simulink model "Stage_4_6_CAN_Fault_Diagnostics_Combined_fault"  (R2025a)
settings: Solver=VariableStepAuto  StartTime=0.0  StopTime=12  RelTol=1e-3
libraries: SignalEditorBlockLib x13, canmsglib x9, simulink x5
settings Model: Creator=sitam  LastModifiedBy=sitam

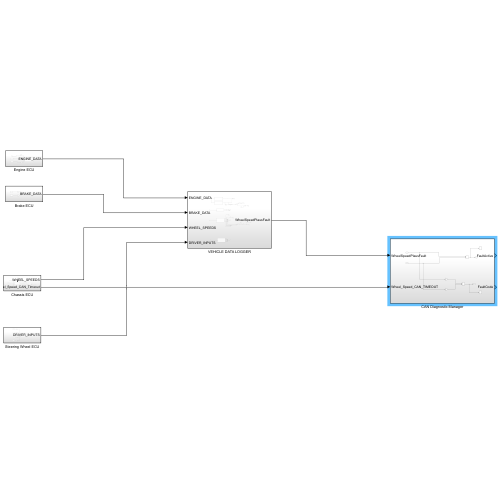
[thumbnail: Simulink's stored preview of the top-level diagram]
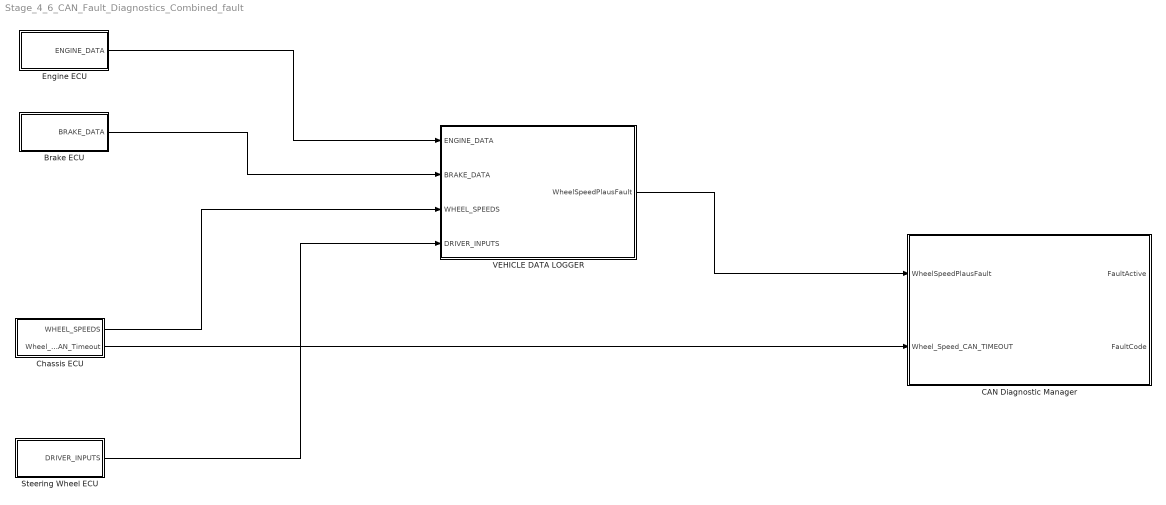
== system Stage_4_6_CAN_Fault_Diagnostics_Combined_fault ==
  Brake ECU : Subsystem
  CAN Diagnostic Manager : Subsystem
  Chassis ECU : Subsystem
  Engine ECU : Subsystem
  Steering Wheel ECU : Subsystem
  VEHICLE DATA LOGGER : Subsystem
  wires:
  Engine ECU/1(ENGINE_DATA) -> VEHICLE DATA LOGGER/1(ENGINE_DATA)
  Brake ECU/1(BRAKE_DATA) -> VEHICLE DATA LOGGER/2(BRAKE_DATA)
  Chassis ECU/1(WHEEL_SPEEDS) -> VEHICLE DATA LOGGER/3(WHEEL_SPEEDS)
  Steering Wheel ECU/1(DRIVER_INPUTS) -> VEHICLE DATA LOGGER/4(DRIVER_INPUTS)
  VEHICLE DATA LOGGER/1(WheelSpeedPlausFault) -> CAN Diagnostic Manager/1(WheelSpeedPlausFault)
  Chassis ECU/2(Wheel_Speed_CAN_Timeout) -> CAN Diagnostic Manager/2(Wheel_Speed_CAN_TIMEOUT)

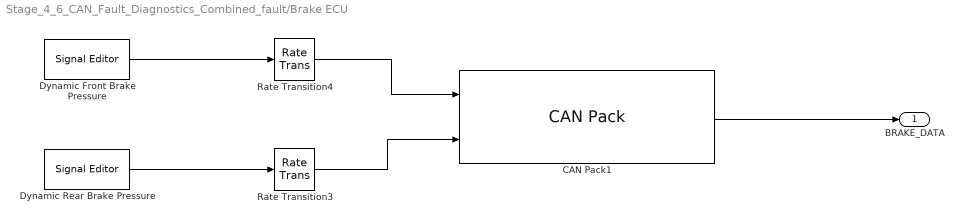
== system Stage_4_6_CAN_Fault_Diagnostics_Combined_fault/Brake ECU ==
  CAN Pack1 : canmsglib/CAN Pack  CANdbFile=C:\Users\sitam\OneDrive\Projects\CAN Bus Project\MotorsportCAN.dbc  MsgList=BRAKE_DATA  MsgName=BRAKE_DATA  MsgIDType=Standard (11-bit identifier)  MsgIdentifier=512  CANIDInput=off  MsgLength=8  Remote=off  ApplyMinMax=off  BusOutput=off  SignalInfo={'FrontBrakePressure','0','16','LE','unsigned','Standard','0','0.01','0','0','200';'RearBrakePressure','16','16','LE','unsigned','Standard','0','0.01','0','0','200'}
      settings: LibrarySourceBlock=canlib/CAN Pack  DataFormat=CANdb specified signals
  Dynamic Front Brake Pressure : SignalEditorBlockLib/Signal Editor  FileName=3_frontbrake.mat  ActiveScenario=Scenario  ActiveSignal=Signal 1  IsBus=off  OutputBusObjectStr=Bus: BusObject  SampleTime=0  ZeroCross=off  OutputAfterFinalValue=Setting to zero  Unit=inherit  PreserveSignalName=on  ApplySigPropsToAllScenarios=on  ApplySigPropsToAllSignals=off  SignalPropertySource=Dialog parameters
  Dynamic Rear Brake Pressure : SignalEditorBlockLib/Signal Editor  FileName=3_rearbrake.mat  ActiveScenario=Scenario  ActiveSignal=Signal 1  IsBus=off  OutputBusObjectStr=Bus: BusObject  SampleTime=0  ZeroCross=off  OutputAfterFinalValue=Setting to zero  Unit=inherit  PreserveSignalName=on  ApplySigPropsToAllScenarios=on  ApplySigPropsToAllSignals=off  SignalPropertySource=Dialog parameters
  Rate Transition3 : RateTransition  OutPortSampleTime=0.01
  Rate Transition4 : RateTransition  OutPortSampleTime=0.01
  BRAKE_DATA : Outport
  wires:
  Rate Transition4/1 -> CAN Pack1/1
  Rate Transition3/1 -> CAN Pack1/2
  CAN Pack1/1 -> BRAKE_DATA/1
  Dynamic Front Brake Pressure/1 -> Rate Transition4/1
  Dynamic Rear Brake Pressure/1 -> Rate Transition3/1

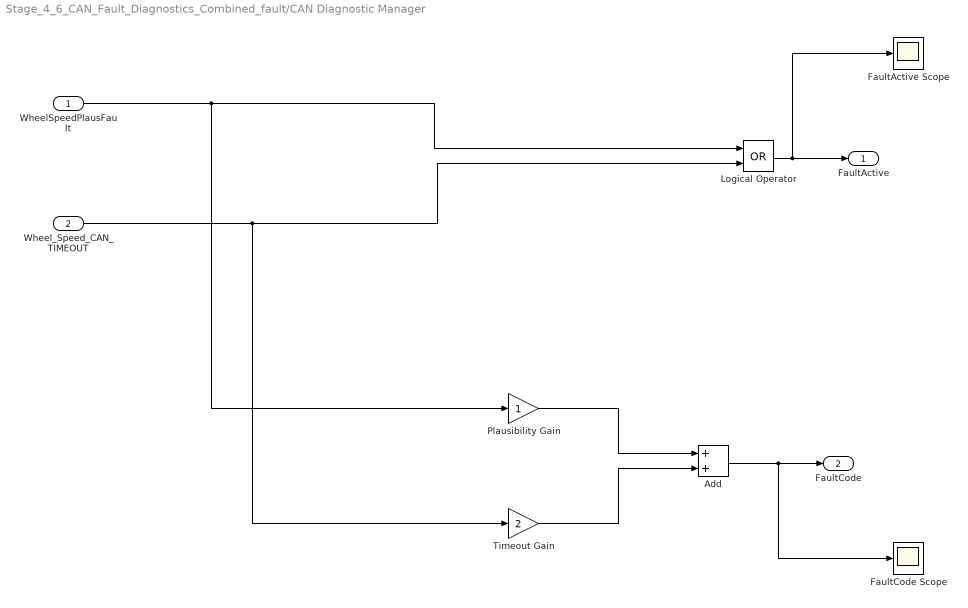
== system Stage_4_6_CAN_Fault_Diagnostics_Combined_fault/CAN Diagnostic Manager ==
  WheelSpeedPlausFault : Inport
  Wheel_Speed_CAN_TIMEOUT : Inport  Port=2
  Add : Sum
  FaultActive Scope : Scope
      settings: ActiveDisplayYMinimum=-0.12499999999999997  ActiveDisplayYMaximum=1.125
  FaultCode Scope : Scope
      settings: ActiveDisplayYMinimum=-0.37499999999999989  ActiveDisplayYMaximum=3.375  DataLoggingVariableName=ScopeData2
  Logical Operator : Logic  Operator=OR  AllPortsSameDT=off  OutDataTypeStr=boolean
  Plausibility Gain : Gain
  Timeout Gain : Gain  Gain=2
  FaultActive : Outport
  FaultCode : Outport  Port=2
  wires:
  WheelSpeedPlausFault/1 -> Plausibility Gain/1, Logical Operator/1
  Wheel_Speed_CAN_TIMEOUT/1 -> Timeout Gain/1, Logical Operator/2
  Logical Operator/1 -> FaultActive Scope/1, FaultActive/1
  Plausibility Gain/1 -> Add/1
  Timeout Gain/1 -> Add/2
  Add/1 -> FaultCode Scope/1, FaultCode/1

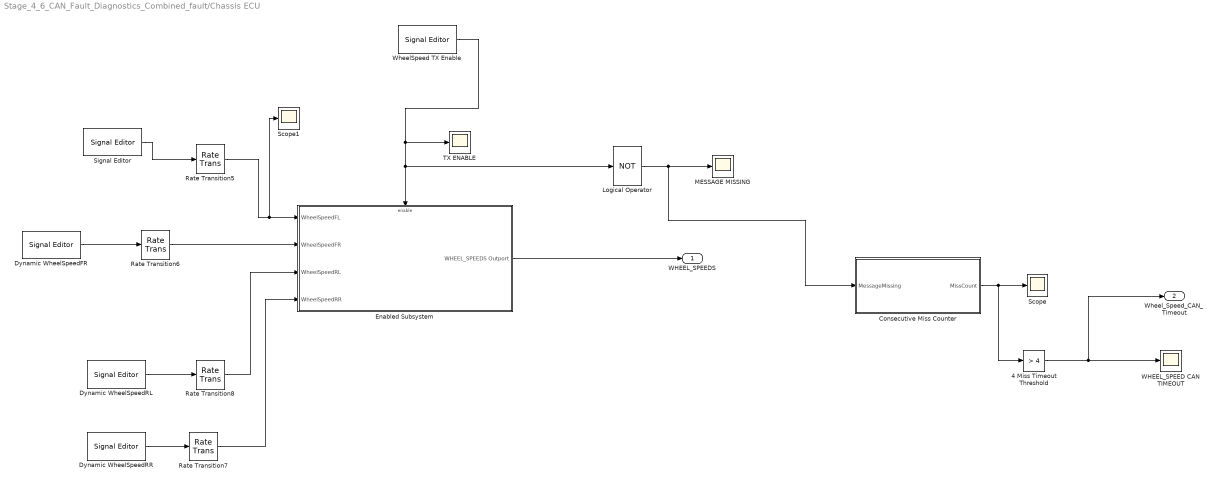
== system Stage_4_6_CAN_Fault_Diagnostics_Combined_fault/Chassis ECU ==
  4 Miss Timeout Threshold : simulink/Logic and Bit Operations/Compare To Constant  relop=>  const=4  OutDataTypeStr=boolean
  Consecutive Miss Counter : Subsystem
  Dynamic WheelSpeedFR : SignalEditorBlockLib/Signal Editor  FileName=3_WheelSpeedFR.mat  ActiveScenario=Scenario  ActiveSignal=Signal 1  IsBus=off  OutputBusObjectStr=Bus: BusObject  SampleTime=0  ZeroCross=off  OutputAfterFinalValue=Setting to zero  Unit=inherit  PreserveSignalName=on  ApplySigPropsToAllScenarios=on  ApplySigPropsToAllSignals=off  SignalPropertySource=Dialog parameters
  Dynamic WheelSpeedRL : SignalEditorBlockLib/Signal Editor  FileName=3_WheelSpeedRL.mat  ActiveScenario=Scenario  ActiveSignal=Signal 1  IsBus=off  OutputBusObjectStr=Bus: BusObject  SampleTime=0  ZeroCross=off  OutputAfterFinalValue=Setting to zero  Unit=inherit  PreserveSignalName=on  ApplySigPropsToAllScenarios=on  ApplySigPropsToAllSignals=off  SignalPropertySource=Dialog parameters
  Dynamic WheelSpeedRR : SignalEditorBlockLib/Signal Editor  FileName=3_WheelSpeedRR.mat  ActiveScenario=Scenario  ActiveSignal=Signal 1  IsBus=off  OutputBusObjectStr=Bus: BusObject  SampleTime=0  ZeroCross=off  OutputAfterFinalValue=Setting to zero  Unit=inherit  PreserveSignalName=on  ApplySigPropsToAllScenarios=on  ApplySigPropsToAllSignals=off  SignalPropertySource=Dialog parameters
  Enabled Subsystem : Subsystem  TreatAsAtomicUnit=on
  Logical Operator : Logic  Operator=NOT  AllPortsSameDT=off  OutDataTypeStr=boolean
  MESSAGE MISSING : Scope
      settings: ActiveDisplayYMinimum=-0.16704928841560512  ActiveDisplayYMaximum=1.2799819615843948  DataLoggingVariableName=ScopeData2
  Rate Transition{5..8} (4 alike) : RateTransition  OutPortSampleTime=0.005
  Scope : Scope
      settings: ActiveDisplayYMinimum=-50.124999999999986  ActiveDisplayYMaximum=451.125  DataLoggingVariableName=ScopeData3
  Scope1 : Scope
      settings: ActiveDisplayYMinimum=7.5000000000000071  ActiveDisplayYMaximum=332.5  DataLoggingVariableName=ScopeData5
  Signal Editor : SignalEditorBlockLib/Signal Editor  FileName=4_6WheelspeedFL.mat  ActiveScenario=Scenario  ActiveSignal=Signal 1  IsBus=off  OutputBusObjectStr=Bus: BusObject  SampleTime=0  ZeroCross=off  OutputAfterFinalValue=Setting to zero  Unit=inherit  PreserveSignalName=on  ApplySigPropsToAllScenarios=on  ApplySigPropsToAllSignals=off  SignalPropertySource=Dialog parameters
  TX ENABLE : Scope
      settings: ActiveDisplayYMinimum=-1  ActiveDisplayYMaximum=1
  WHEEL_SPEED CAN TIMEOUT : Scope
      settings: ActiveDisplayYMinimum=-0.12499999999999997  ActiveDisplayYMaximum=1.125  DataLoggingVariableName=ScopeData4
  WheelSpeed TX Enable : SignalEditorBlockLib/Signal Editor  FileName=4_6WHEEL_SPEEDS_Tx_Enable.mat  ActiveScenario=Scenario  ActiveSignal=Signal 1  IsBus=off  OutputBusObjectStr=Bus: BusObject  SampleTime=0  ZeroCross=off  OutputAfterFinalValue=Setting to zero  Unit=inherit  PreserveSignalName=on  ApplySigPropsToAllScenarios=on  ApplySigPropsToAllSignals=off  SignalPropertySource=Dialog parameters
  WHEEL_SPEEDS : Outport
  Wheel_Speed_CAN_Timeout : Outport  Port=2
  wires:
  Rate Transition8/1 -> Enabled Subsystem/3(WheelSpeedRL)
  Enabled Subsystem/1(WHEEL_SPEEDS Outport) -> WHEEL_SPEEDS/1
  Dynamic WheelSpeedFR/1 -> Rate Transition6/1
  Dynamic WheelSpeedRL/1 -> Rate Transition8/1
  Rate Transition5/1 -> Scope1/1, Enabled Subsystem/1(WheelSpeedFL)
  Dynamic WheelSpeedRR/1 -> Rate Transition7/1
  Rate Transition7/1 -> Enabled Subsystem/4(WheelSpeedRR)
  Rate Transition6/1 -> Enabled Subsystem/2(WheelSpeedFR)
  Logical Operator/1 -> Consecutive Miss Counter/1(MessageMissing), MESSAGE MISSING/1
  Consecutive Miss Counter/1(MissCount) -> 4 Miss Timeout Threshold/1, Scope/1
  4 Miss Timeout Threshold/1 -> Wheel_Speed_CAN_Timeout/1, WHEEL_SPEED CAN TIMEOUT/1
  Signal Editor/1 -> Rate Transition5/1
  WheelSpeed TX Enable/1 -> TX ENABLE/1, Enabled Subsystem/Enable, Logical Operator/1

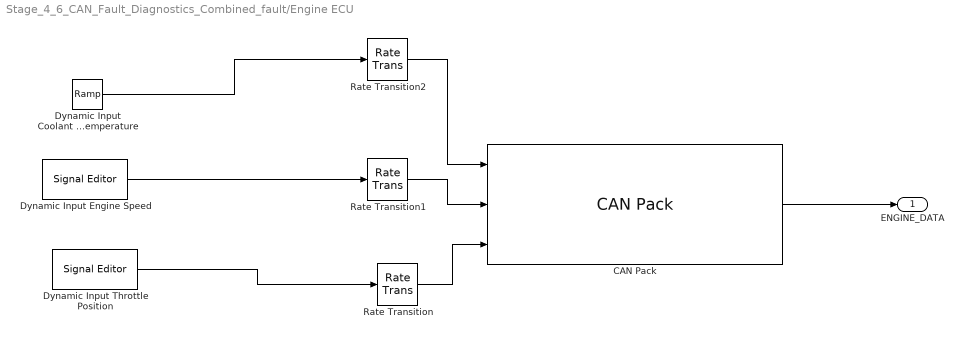
== system Stage_4_6_CAN_Fault_Diagnostics_Combined_fault/Engine ECU ==
  CAN Pack : canmsglib/CAN Pack  CANdbFile=C:\Users\sitam\OneDrive\Projects\CAN Bus Project\MotorsportCAN.dbc  MsgList=ENGINE_DATA  MsgName=ENGINE_DATA  MsgIDType=Standard (11-bit identifier)  MsgIdentifier=256  CANIDInput=off  MsgLength=8  Remote=off  ApplyMinMax=off  BusOutput=off  SignalInfo={'CoolantTemperature','24','8','LE','unsigned','Standard','0','1','-40','-40','150';'EngineSpeed','0','16','LE','unsigned','Standard','0','0.25','0','0','15000';'ThrottlePosition','16','8','LE','unsigned','Standard','0','0.4','0','0','100'}
      settings: LibrarySourceBlock=canlib/CAN Pack  DataFormat=CANdb specified signals
  Dynamic Input Coolant Temperature : simulink/Sources/Ramp  slope=1  start=0  InitialOutput=85
  Dynamic Input Engine Speed : SignalEditorBlockLib/Signal Editor  FileName=2_2-enginespeed.mat  ActiveScenario=Scenario  ActiveSignal=Signal 1  IsBus=off  OutputBusObjectStr=Bus: BusObject  SampleTime=0  ZeroCross=off  OutputAfterFinalValue=Setting to zero  Unit=inherit  PreserveSignalName=on  ApplySigPropsToAllScenarios=on  ApplySigPropsToAllSignals=off  SignalPropertySource=Dialog parameters
  Dynamic Input Throttle Position : SignalEditorBlockLib/Signal Editor  FileName=2_2-throttlepos.mat  ActiveScenario=Scenario  ActiveSignal=Signal 1  IsBus=off  OutputBusObjectStr=Bus: BusObject  SampleTime=0  ZeroCross=off  OutputAfterFinalValue=Setting to zero  Unit=inherit  PreserveSignalName=on  ApplySigPropsToAllScenarios=on  ApplySigPropsToAllSignals=off  SignalPropertySource=Dialog parameters
  Rate Transition : RateTransition  OutPortSampleTime=0.01
  Rate Transition1 : RateTransition  OutPortSampleTime=0.01
  Rate Transition2 : RateTransition  OutPortSampleTime=0.01
  ENGINE_DATA : Outport
  wires:
  CAN Pack/1 -> ENGINE_DATA/1
  Dynamic Input Coolant Temperature/1 -> Rate Transition2/1
  Rate Transition2/1 -> CAN Pack/1
  Dynamic Input Engine Speed/1 -> Rate Transition1/1
  Rate Transition1/1 -> CAN Pack/2
  Dynamic Input Throttle Position/1 -> Rate Transition/1
  Rate Transition/1 -> CAN Pack/3

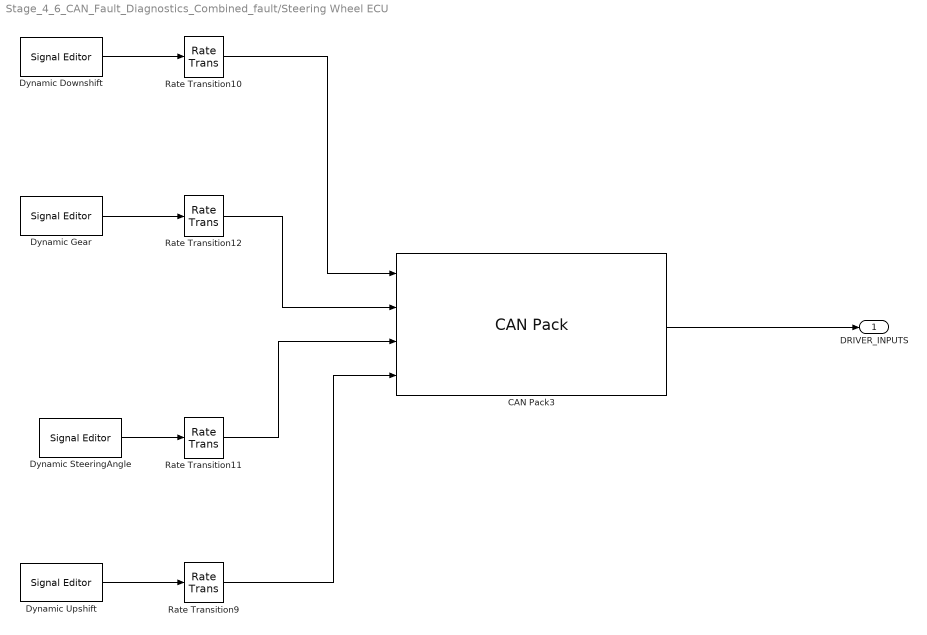
== system Stage_4_6_CAN_Fault_Diagnostics_Combined_fault/Steering Wheel ECU ==
  CAN Pack3 : canmsglib/CAN Pack  CANdbFile=C:\Users\sitam\OneDrive\Projects\CAN Bus Project\MotorsportCAN.dbc  MsgList=DRIVER_INPUTS  MsgName=DRIVER_INPUTS  MsgIDType=Standard (11-bit identifier)  MsgIdentifier=1024  CANIDInput=off  MsgLength=8  Remote=off  ApplyMinMax=off  BusOutput=off  SignalInfo={'Downshift','25','1','LE','unsigned','Standard','0','1','0','0','1';'Gear','16','3','LE','unsigned','Standard','0','1','0','0','7';'SteeringAngle','0','16','LE','signed','Standard','0','0.1','0','-540','540';'Upshift','24','1','LE','unsigned','Standard','0','1','0','0','1'}
      settings: LibrarySourceBlock=canlib/CAN Pack  DataFormat=CANdb specified signals
  Dynamic Downshift : SignalEditorBlockLib/Signal Editor  FileName=3_downshift.mat  ActiveScenario=Scenario  ActiveSignal=Signal 1  IsBus=off  OutputBusObjectStr=Bus: BusObject  SampleTime=0  ZeroCross=off  OutputAfterFinalValue=Setting to zero  Unit=inherit  PreserveSignalName=on  ApplySigPropsToAllScenarios=on  ApplySigPropsToAllSignals=off  SignalPropertySource=Dialog parameters
  Dynamic Gear : SignalEditorBlockLib/Signal Editor  FileName=3_gear.mat  ActiveScenario=Scenario  ActiveSignal=Signal 1  IsBus=off  OutputBusObjectStr=Bus: BusObject  SampleTime=0  ZeroCross=off  OutputAfterFinalValue=Setting to zero  Unit=inherit  PreserveSignalName=on  ApplySigPropsToAllScenarios=on  ApplySigPropsToAllSignals=off  SignalPropertySource=Dialog parameters
  Dynamic SteeringAngle : SignalEditorBlockLib/Signal Editor  FileName=3_steeringangle.mat  ActiveScenario=Scenario  ActiveSignal=Signal 1  IsBus=off  OutputBusObjectStr=Bus: BusObject  SampleTime=0  ZeroCross=off  OutputAfterFinalValue=Setting to zero  Unit=inherit  PreserveSignalName=on  ApplySigPropsToAllScenarios=on  ApplySigPropsToAllSignals=off  SignalPropertySource=Dialog parameters
  Dynamic Upshift : SignalEditorBlockLib/Signal Editor  FileName=3_upshift.mat  ActiveScenario=Scenario  ActiveSignal=Signal 1  IsBus=off  OutputBusObjectStr=Bus: BusObject  SampleTime=0  ZeroCross=off  OutputAfterFinalValue=Setting to zero  Unit=inherit  PreserveSignalName=on  ApplySigPropsToAllScenarios=on  ApplySigPropsToAllSignals=off  SignalPropertySource=Dialog parameters
  Rate Transition{9..12} (4 alike) : RateTransition  OutPortSampleTime=0.02
  DRIVER_INPUTS : Outport
  wires:
  Rate Transition10/1 -> CAN Pack3/1
  Dynamic Upshift/1 -> Rate Transition9/1
  Rate Transition11/1 -> CAN Pack3/3
  Dynamic SteeringAngle/1 -> Rate Transition11/1
  Rate Transition9/1 -> CAN Pack3/4
  Rate Transition12/1 -> CAN Pack3/2
  Dynamic Gear/1 -> Rate Transition12/1
  Dynamic Downshift/1 -> Rate Transition10/1
  CAN Pack3/1 -> DRIVER_INPUTS/1

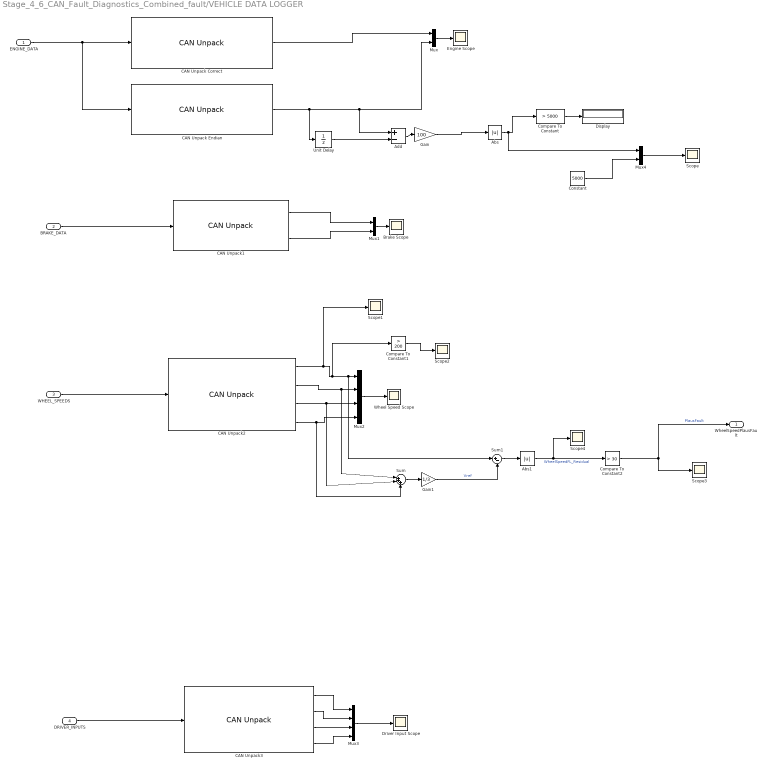
== system Stage_4_6_CAN_Fault_Diagnostics_Combined_fault/VEHICLE DATA LOGGER ==
  ENGINE_DATA : Inport
  BRAKE_DATA : Inport  Port=2
  WHEEL_SPEEDS : Inport  Port=3
  DRIVER_INPUTS : Inport  Port=4
  Abs : Abs  SaturateOnIntegerOverflow=off
  Abs1 : Abs  SaturateOnIntegerOverflow=off
  Add : Sum  Inputs=+-
  Brake Scope : Scope
      settings: ActiveDisplayYMinimum=-1  ActiveDisplayYMaximum=1  DataLoggingVariableName=ScopeData15
  CAN Unpack Correct : canmsglib/CAN Unpack  CANdbFile=C:\Users\sitam\OneDrive\Projects\CAN Bus Project\MotorsportCAN.dbc  MsgList=ENGINE_DATA  MsgName=ENGINE_DATA  MsgIDType=Standard (11-bit identifier)  MsgIdentifier=256  MsgLength=8  SignalInfo={'CoolantTemperature','24','8','LE','unsigned','Standard','0','1','-40','-40','150';'EngineSpeed','0','16','LE','unsigned','Standard','0','0.25','0','0','15000';'ThrottlePosition','16','8','LE','unsigned','Standard','0','0.4','0','0','100'}  IDPort=off  TimestampPort=off  ErrorPort=off  RemotePort=off  LengthPort=off  StatusPort=off  ApplyMinMax=off
      settings: LibrarySourceBlock=canlib/CAN Unpack  DataFormat=CANdb specified signals
  CAN Unpack Endian : canmsglib/CAN Unpack  CANdbFile=C:\Users\sitam\OneDrive\Projects\CAN Bus Project\dbc files\MotorsportCAN_Fault_Endian.dbc  MsgList=ENGINE_DATA  MsgName=ENGINE_DATA  MsgIDType=Standard (11-bit identifier)  MsgIdentifier=256  MsgLength=8  SignalInfo={'CoolantTemperature','24','8','LE','unsigned','Standard','0','1','-40','-40','150';'EngineSpeed','8','16','BE','unsigned','Standard','0','0.25','0','0','15000';'ThrottlePosition','16','8','LE','unsigned','Standard','0','0.4','0','0','100'}  IDPort=off  TimestampPort=off  ErrorPort=off  RemotePort=off  LengthPort=off  StatusPort=off  ApplyMinMax=off
      settings: LibrarySourceBlock=canlib/CAN Unpack  DataFormat=CANdb specified signals
  CAN Unpack1 : canmsglib/CAN Unpack  CANdbFile=C:\Users\sitam\OneDrive\Projects\CAN Bus Project\MotorsportCAN.dbc  MsgList=BRAKE_DATA  MsgName=BRAKE_DATA  MsgIDType=Standard (11-bit identifier)  MsgIdentifier=512  MsgLength=8  SignalInfo={'FrontBrakePressure','0','16','LE','unsigned','Standard','0','0.01','0','0','200';'RearBrakePressure','16','16','LE','unsigned','Standard','0','0.01','0','0','200'}  IDPort=off  TimestampPort=off  ErrorPort=off  RemotePort=off  LengthPort=off  StatusPort=off  ApplyMinMax=off
      settings: LibrarySourceBlock=canlib/CAN Unpack  DataFormat=CANdb specified signals
  CAN Unpack2 : canmsglib/CAN Unpack  CANdbFile=C:\Users\sitam\OneDrive\Projects\CAN Bus Project\MotorsportCAN.dbc  MsgList=WHEEL_SPEEDS  MsgName=WHEEL_SPEEDS  MsgIDType=Standard (11-bit identifier)  MsgIdentifier=768  MsgLength=8  SignalInfo={'WheelSpeedFL','0','16','LE','unsigned','Standard','0','0.01','0','0','350';'WheelSpeedFR','16','16','LE','unsigned','Standard','0','0.01','0','0','350';'WheelSpeedRL','32','16','LE','unsigned','Standard','0','0.01','0','0','350';'WheelSpeedRR','48','16','LE','unsigned','Standard','0','0.01','0','0','350'}  IDPort=off  TimestampPort=off  ErrorPort=off  RemotePort=off  LengthPort=off  StatusPort=off  ApplyMinMax=off
      settings: LibrarySourceBlock=canlib/CAN Unpack  DataFormat=CANdb specified signals
  CAN Unpack3 : canmsglib/CAN Unpack  CANdbFile=C:\Users\sitam\OneDrive\Projects\CAN Bus Project\MotorsportCAN.dbc  MsgList=DRIVER_INPUTS  MsgName=DRIVER_INPUTS  MsgIDType=Standard (11-bit identifier)  MsgIdentifier=1024  MsgLength=8  SignalInfo={'Downshift','25','1','LE','unsigned','Standard','0','1','0','0','1';'Gear','16','3','LE','unsigned','Standard','0','1','0','0','7';'SteeringAngle','0','16','LE','signed','Standard','0','0.1','0','-540','540';'Upshift','24','1','LE','unsigned','Standard','0','1','0','0','1'}  IDPort=off  TimestampPort=off  ErrorPort=off  RemotePort=off  LengthPort=off  StatusPort=off  ApplyMinMax=off
      settings: LibrarySourceBlock=canlib/CAN Unpack  DataFormat=CANdb specified signals
  Compare To Constant : simulink/Logic and Bit Operations/Compare To Constant  relop=>  const=5000  OutDataTypeStr=boolean
  Compare To Constant1 : simulink/Logic and Bit Operations/Compare To Constant  relop=>  const=200  OutDataTypeStr=boolean
  Compare To Constant2 : simulink/Logic and Bit Operations/Compare To Constant  relop=>  const=30  OutDataTypeStr=boolean
  Constant : Constant  Value=5000
  Display : Display
  Driver Input Scope : Scope
      settings: ActiveDisplayYMinimum=-149.00944352064721  ActiveDisplayYMaximum=158.80440759196159  DataLoggingVariableName=ScopeData13
  Engine Scope : Scope
      settings: ActiveDisplayYMinimum=-11017.645713138911  ActiveDisplayYMaximum=31195.36696654859  DataLoggingVariableName=ScopeData16
  Gain : Gain  Gain=100
  Gain1 : Gain  Gain=1/3
  Mux : Mux  Inputs=2
  Mux1 : Mux  Inputs=2
  Mux2 : Mux
  Mux3 : Mux
  Mux4 : Mux  Inputs=2
  Scope{,1..4} (5 alike) : Scope
      Scope settings: ActiveDisplayYMinimum=-173718.74999999997  ActiveDisplayYMaximum=1.61346875E+6
      Scope1 settings: ActiveDisplayYMinimum=-1  ActiveDisplayYMaximum=1  DataLoggingVariableName=ScopeData6
      Scope2 settings: ActiveDisplayYMinimum=-1  ActiveDisplayYMaximum=1  DataLoggingVariableName=ScopeData8
      Scope3 settings: ActiveDisplayYMinimum=-0.12499999999999997  ActiveDisplayYMaximum=1.125  DataLoggingVariableName=ScopeData9
      Scope4 settings: ActiveDisplayYMinimum=-27.499999999999993  ActiveDisplayYMaximum=247.5  DataLoggingVariableName=ScopeData10
  Sum : Sum  Inputs=|+++
  Sum1 : Sum  Inputs=|+-
  Unit Delay : UnitDelay  SampleTime=0.01  HasFrameUpgradeWarning=on
  Wheel Speed Scope : Scope
      settings: ActiveDisplayYMinimum=33.586083369518022  ActiveDisplayYMaximum=140.72894051237517  DataLoggingVariableName=ScopeData14
  WheelSpeedPlausFault : Outport
  wires:
  ENGINE_DATA/1 -> CAN Unpack Endian/1, CAN Unpack Correct/1
  DRIVER_INPUTS/1 -> CAN Unpack3/1
  WHEEL_SPEEDS/1 -> CAN Unpack2/1
  BRAKE_DATA/1 -> CAN Unpack1/1
  CAN Unpack1/1 -> Mux1/1
  CAN Unpack1/2 -> Mux1/2
  CAN Unpack2/1 -> Scope1/1, Compare To Constant1/1, Sum1/1, Mux2/1
  CAN Unpack2/2 -> Sum/1, Mux2/2
  CAN Unpack2/3 -> Sum/2, Mux2/3
  CAN Unpack2/4 -> Sum/3, Mux2/4
  CAN Unpack3/1 -> Mux3/1
  CAN Unpack3/2 -> Mux3/2
  CAN Unpack3/3 -> Mux3/3
  CAN Unpack3/4 -> Mux3/4
  Mux3/1 -> Driver Input Scope/1
  Mux2/1 -> Wheel Speed Scope/1
  Mux1/1 -> Brake Scope/1
  Mux/1 -> Engine Scope/1
  CAN Unpack Endian/2 -> Unit Delay/1, Add/1, Mux/2
  CAN Unpack Correct/2 -> Mux/1
  Abs/1 -> Mux4/1, Compare To Constant/1
  Compare To Constant/1 -> Display/1
  Add/1 -> Gain/1
  Gain/1 -> Abs/1
  Unit Delay/1 -> Add/2
  Constant/1 -> Mux4/2
  Mux4/1 -> Scope/1
  Compare To Constant1/1 -> Scope2/1
  Sum/1 -> Gain1/1
  Gain1/1 -> Sum1/2  "Vref"
  Sum1/1 -> Abs1/1
  Abs1/1 -> Scope4/1, Compare To Constant2/1  "WheelSpeedFL_Residual"
  Compare To Constant2/1 -> WheelSpeedPlausFault/1, Scope3/1  "PlausFault"

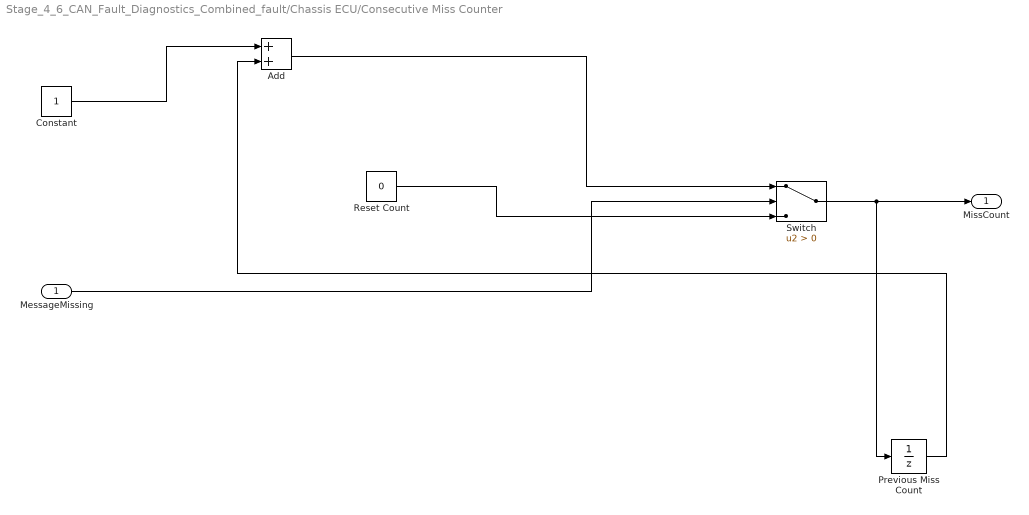
== system Stage_4_6_CAN_Fault_Diagnostics_Combined_fault/Chassis ECU/Consecutive Miss Counter ==
  MessageMissing : Inport
  Add : Sum
  Constant : Constant
  Previous Miss Count : UnitDelay  SampleTime=0.005  HasFrameUpgradeWarning=on
  Reset Count : Constant  Value=0
  Switch : Switch  Criteria=u2 > Threshold  SaturateOnIntegerOverflow=off  InputSameDT=off
  MissCount : Outport
  wires:
  Constant/1 -> Add/1
  Switch/1 -> Previous Miss Count/1, MissCount/1
  Previous Miss Count/1 -> Add/2
  Add/1 -> Switch/1
  MessageMissing/1 -> Switch/2
  Reset Count/1 -> Switch/3

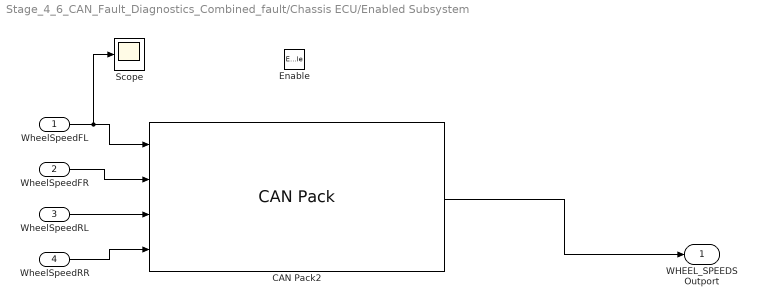
== system Stage_4_6_CAN_Fault_Diagnostics_Combined_fault/Chassis ECU/Enabled Subsystem ==
  WheelSpeedFL : Inport
  WheelSpeedFR : Inport  Port=2
  WheelSpeedRL : Inport  Port=3
  WheelSpeedRR : Inport  Port=4
  Enable : EnablePort
  CAN Pack2 : canmsglib/CAN Pack  CANdbFile=C:\Users\sitam\OneDrive\Projects\CAN Bus Project\MotorsportCAN.dbc  MsgList=WHEEL_SPEEDS  MsgName=WHEEL_SPEEDS  MsgIDType=Standard (11-bit identifier)  MsgIdentifier=768  CANIDInput=off  MsgLength=8  Remote=off  ApplyMinMax=off  BusOutput=off  SignalInfo={'WheelSpeedFL','0','16','LE','unsigned','Standard','0','0.01','0','0','350';'WheelSpeedFR','16','16','LE','unsigned','Standard','0','0.01','0','0','350';'WheelSpeedRL','32','16','LE','unsigned','Standard','0','0.01','0','0','350';'WheelSpeedRR','48','16','LE','unsigned','Standard','0','0.01','0','0','350'}
      settings: LibrarySourceBlock=canlib/CAN Pack  DataFormat=CANdb specified signals
  Scope : Scope
      settings: ActiveDisplayYMinimum=28.750000000000004  ActiveDisplayYMaximum=141.25  DataLoggingVariableName=ScopeData7
  WHEEL_SPEEDS Outport : Outport
  wires:
  WheelSpeedFL/1 -> Scope/1, CAN Pack2/1
  WheelSpeedFR/1 -> CAN Pack2/2
  WheelSpeedRL/1 -> CAN Pack2/3
  WheelSpeedRR/1 -> CAN Pack2/4
  CAN Pack2/1 -> WHEEL_SPEEDS Outport/1
